simulink model "myTMSI"  (R2017b)
settings: Solver=FixedStepAuto  StartTime=0.0  StopTime=Inf  FixedStep=0.01  RelTol=1e-3
StopFcn:
  | [file,path] = uiputfile;
  | cd(path)
  | save(file, 'EMGdata', 'EMGcount', 'QuatAngle', 'Angles', 'Angles23', 'QuatAngle1')
  | cd ..
libraries: dspindex x16
settings Model: SimulationMode=external  ExtModeTrigDuration=50000  Creator=constantin  LastModifiedBy=root
settings DataIOCC: SaveFormat=Array
settings OptimizationCC: ExpressionDepthLimit=2147483647  LifeSpan=1
settings DebuggingCC: UnderspecifiedInitializationDetection=Classic  MergeDetectMultiDrivingBlocksExec=none  SolverPrmCheckMsg=warning  StateNameClashWarn=warning  SFUnexpectedBacktrackingDiag=warning  SFNoUnconditionalDefaultTransitionDiag=warning  SFExecutionAtInitializationDiag=none
settings HardwareCC: ProdBitPerPointer=32  ProdBitPerSizeT=32  ProdBitPerPtrDiffT=32  ProdLargestAtomicFloat=None  ProdIntDivRoundTo=Undefined  ProdEndianess=Unspecified  ProdWordSize=32  ProdHWDeviceType=32-bit Generic
settings ModelReferenceCC: PropagateSignalLabelsOutOfModel=off
settings SFSimCC: MATLABDynamicMemAlloc=off
settings RTWCC: SystemTargetFile=ert_linux.tlc  MakeCommand=make_rtw OPTS=-DWITH_HW OPTIMIZATION_FLAGS=-O3  TemplateMakefile=ert_linux.tmf  Description=Linux Embedded Coder  TargetLang=C++
settings CodeAppCC: IgnoreCustomStorageClasses=off  CustomSymbolStrType=$N$R$M  StateflowObjectComments=on  InternalIdentifier=Classic
settings STFCustomTargetCC: ModelReferenceCompliant=off  CombineOutputUpdateFcns=on  ERTCustomFileBanners=on  SupportComplex=off  RemoveResetFunc=on  SupportVariableSizeSignals=on  MATLABClassNameForMDSCustomization=Simulink.SoftwareTarget.ERTCustomization  GRTInterface=off  SystemTargetFile=ert_linux.tlc
settings ERTTargetCC: MultiwordLength=2048  ModelReferenceCompliant=off  ParMdlRefBuildCompliant=off  CompOptLevelCompliant=off  ConcurrentExecutionCompliant=off  SupportComplex=off  SupportContinuousTime=on  SupportNonInlinedSFcns=on  SupportVariableSizeSignals=on  ModelStepFunctionPrototypeControlCompliant=off  CPPClassGenCompliant=off  UseToolchainInfoCompliant=off  ExtMode=on  ExtModeMexArgs='127.0.0.1' 1 17725  MultiInstanceErrorCode=None  ERTCustomFileTemplate=ert_linux_file_process.tlc  ConvertIfToSwitch=off  SuppressUnreachableDefaultCases=off
settings ConfigComp: CovMetricSettings=dw  CovHtmlReporting=on  CovSaveCumulativeToWorkspaceVar=on  CovSaveSingleToWorkspaceVar=on  CovExternalEMLEnable=off  CovSFcnEnable=off
settings SimscapeCC: SimscapeNormalizeSystem=off
settings ConfigurationSet: Description=SimMechanics 2G

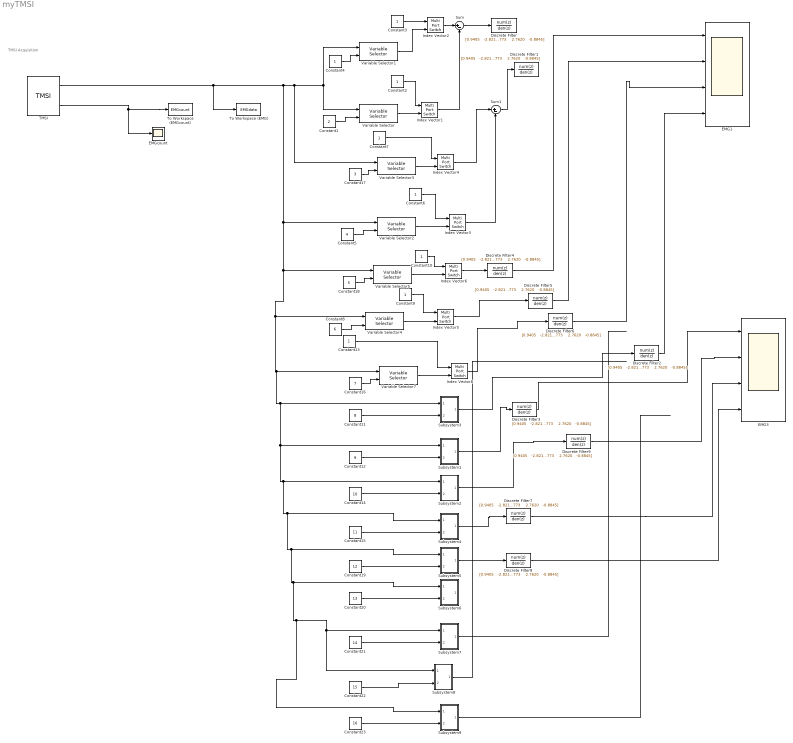
== system myTMSI ==
  note: TMSI Acquisition
  Constant1 : Constant  Value=2
  Constant{2..4,6..7,9..10,13} (8 alike) : Constant
  Constant11 : Constant  Value=8
  Constant12 : Constant  Value=9
  Constant14 : Constant  Value=10
  Constant15 : Constant  Value=11
  Constant16 : Constant  Value=7
  Constant17 : Constant  Value=3
  Constant18 : Constant  Value=5
  Constant19 : Constant  Value=12
  Constant20 : Constant  Value=13
  Constant21 : Constant  Value=14
  Constant22 : Constant  Value=15
  Constant23 : Constant  Value=16
  Constant5 : Constant  Value=4
  Constant8 : Constant  Value=6
  Discrete Filter : DiscreteFilter  Numerator=|  Denominator="[1.0000   -2.8773    2.7620   -0.8845]"
      | [0.9405   -2.8214    2.8214   -0.9405
      | ]
  Discrete Filter{1..9} (9 alike) : DiscreteFilter  Numerator="[0.9405   -2.8214    2.8214   -0.9405]"  Denominator="[1.0000   -2.8773    2.7620   -0.8845]"
  EMG1 : Scope  NumInputPorts=4
  EMG3 : Scope  NumInputPorts=4
  EMGcount : Scope
  Index Vector{1..6,8} (7 alike) : MultiPortSwitch  DataPortOrder=Zero-based contiguous  Inputs=1  zeroidx=on
  Subsystem1 : Subsystem
  Subsystem2 : Subsystem
  Subsystem3 : Subsystem
  Subsystem4 : Subsystem
  Subsystem5 : Subsystem
  Subsystem6 : Subsystem
  Subsystem7 : Subsystem
  Subsystem8 : Subsystem
  Subsystem9 : Subsystem
  Sum : Sum  Inputs=|+-
  Sum1 : Sum  Inputs=|+-
  TMSI : S-Function  FunctionName=TMSI  Parameters=uint16(frequency) int32(aux) int32(digital) int32(vectorsize) int32(ch)  SFunctionDeploymentMode=off  EnableBusSupport=off  mask{frequency=1, ch=[1 2 3 4 17 18 19 20 21 22 23 24 25 26 27 28], vectorsize=20, aux=29, digital=30}
      mask prompts: frequency "Please select a frequency"; ch "Please enter an array for channels e.g [17 29]"; vectorsize "Please enter the vector output size"; aux "Please enter the aux channel"; digital "Please enter digital channel"
      mask DialogControl DescTextVar Prompt: TMSI Block for EMG measurement
      mask Display:
      | disp('TMSI')
      | port_label('output', 1, 'data')
      | port_label('output', 2, 'status')
  To Workspace (EMG) : ToWorkspace  VariableName=EMGdata  SaveFormat=Structure With Time  SampleTime=-1
  To Workspace (EMGcount) : ToWorkspace  VariableName=EMGcount  SaveFormat=Structure With Time  SampleTime=-1
  Variable Selector{,1..5,7} (7 alike) : dspindex/Variable Selector  NumInputs=1  rowsOrCols=Rows  IdxMode=Variable  Elements=[1 3]  ZerOneIdxMode=One-based  errmode=Clip Index  FillMode=on  FillValues=0
  wires:
  TMSI/2 -> To Workspace (EMGcount)/1, EMGcount/1
  Constant1/1 -> Variable Selector/2
  Variable Selector/1 -> Index Vector1/2
  Constant2/1 -> Index Vector1/1
  Variable Selector1/1 -> Index Vector2/2
  Constant3/1 -> Index Vector2/1
  Constant4/1 -> Variable Selector1/2
  Variable Selector2/1 -> Index Vector3/2
  Constant6/1 -> Index Vector3/1
  Variable Selector3/1 -> Index Vector4/2
  Constant7/1 -> Index Vector4/1
  Constant5/1 -> Variable Selector2/2
  Constant17/1 -> Variable Selector3/2
  Index Vector6/1 -> Discrete Filter4/1
  Variable Selector4/1 -> Index Vector5/2
  Constant9/1 -> Index Vector5/1
  Variable Selector5/1 -> Index Vector6/2
  Constant10/1 -> Index Vector6/1
  Constant8/1 -> Variable Selector4/2
  Constant18/1 -> Variable Selector5/2
  Index Vector5/1 -> Discrete Filter5/1
  Index Vector8/1 -> Discrete Filter6/1
  Variable Selector7/1 -> Index Vector8/2
  Constant13/1 -> Index Vector8/1
  Constant16/1 -> Variable Selector7/2
  Index Vector4/1 -> Sum1/1
  Index Vector3/1 -> Sum1/2
  TMSI/1 -> To Workspace (EMG)/1, Subsystem3/1(In1), Subsystem9/1(In1), Subsystem7/1(In1), Subsystem8/1(In1), Subsystem6/1(In1), Subsystem5/1(In1), Subsystem4/1(In1), Subsystem2/1(In1), Subsystem1/1(In1), Variable Selector7/1, Variable Selector4/1, Variable Selector5/1, Variable Selector2/1, Variable Selector3/1, Variable Selector1/1, Variable Selector/1
  Index Vector2/1 -> Sum/1
  Index Vector1/1 -> Sum/2
  Sum/1 -> Discrete Filter/1
  Sum1/1 -> Discrete Filter1/1
  Discrete Filter4/1 -> EMG1/1
  Discrete Filter5/1 -> EMG1/2
  Discrete Filter6/1 -> EMG1/3
  Constant11/1 -> Subsystem3/2(In2)
  Subsystem3/1(Out1) -> Discrete Filter2/1
  Constant12/1 -> Subsystem1/2(In2)
  Constant14/1 -> Subsystem2/2(In2)
  Constant19/1 -> Subsystem5/2(In2)
  Constant15/1 -> Subsystem4/2(In2)
  Constant20/1 -> Subsystem6/2(In2)
  Constant21/1 -> Subsystem7/2(In2)
  Constant22/1 -> Subsystem8/2(In2)
  Constant23/1 -> Subsystem9/2(In2)
  Subsystem7/1(Out1) -> ?
  Subsystem8/1(Out1) -> ?
  Subsystem9/1(Out1) -> ?
  Discrete Filter2/1 -> EMG1/4
  Subsystem1/1(Out1) -> Discrete Filter3/1
  Discrete Filter3/1 -> EMG3/1
  Subsystem2/1(Out1) -> Discrete Filter9/1
  Subsystem4/1(Out1) -> Discrete Filter7/1
  Subsystem5/1(Out1) -> Discrete Filter8/1
  Discrete Filter9/1 -> EMG3/2
  Discrete Filter7/1 -> EMG3/3
  Discrete Filter8/1 -> EMG3/4

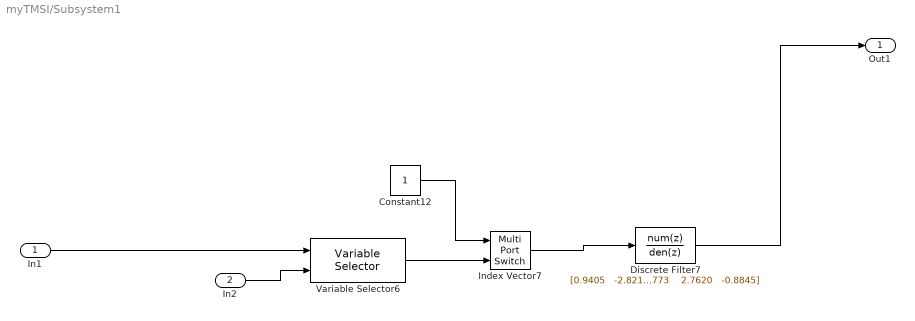
== system myTMSI/Subsystem1 ==
  In1 : Inport
  In2 : Inport  Port=2
  Constant12 : Constant
  Discrete Filter7 : DiscreteFilter  Numerator="[0.9405   -2.8214    2.8214   -0.9405]"  Denominator="[1.0000   -2.8773    2.7620   -0.8845]"
  Index Vector7 : MultiPortSwitch  DataPortOrder=Zero-based contiguous  Inputs=1  zeroidx=on
  Variable Selector6 : dspindex/Variable Selector  NumInputs=1  rowsOrCols=Rows  IdxMode=Variable  Elements=[1 3]  ZerOneIdxMode=One-based  errmode=Clip Index  FillMode=on  FillValues=0
  Out1 : Outport
  wires:
  In1/1 -> Variable Selector6/1
  Discrete Filter7/1 -> Out1/1
  Variable Selector6/1 -> Index Vector7/2
  Constant12/1 -> Index Vector7/1
  In2/1 -> Variable Selector6/2
  Index Vector7/1 -> Discrete Filter7/1

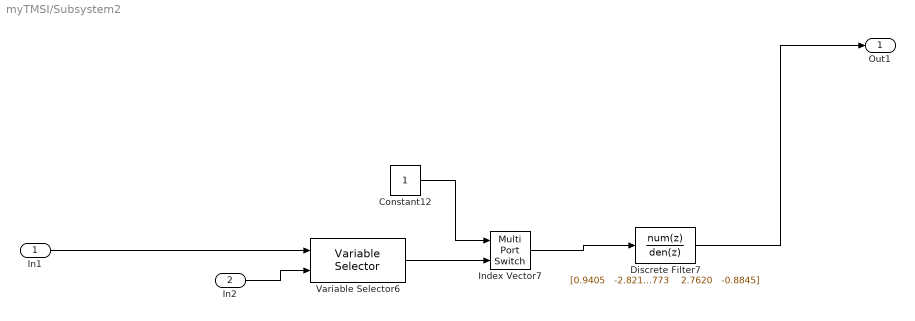
== system myTMSI/Subsystem2 ==
  In1 : Inport
  In2 : Inport  Port=2
  Constant12 : Constant
  Discrete Filter7 : DiscreteFilter  Numerator="[0.9405   -2.8214    2.8214   -0.9405]"  Denominator="[1.0000   -2.8773    2.7620   -0.8845]"
  Index Vector7 : MultiPortSwitch  DataPortOrder=Zero-based contiguous  Inputs=1  zeroidx=on
  Variable Selector6 : dspindex/Variable Selector  NumInputs=1  rowsOrCols=Rows  IdxMode=Variable  Elements=[1 3]  ZerOneIdxMode=One-based  errmode=Clip Index  FillMode=on  FillValues=0
  Out1 : Outport
  wires:
  In1/1 -> Variable Selector6/1
  Discrete Filter7/1 -> Out1/1
  Variable Selector6/1 -> Index Vector7/2
  Constant12/1 -> Index Vector7/1
  In2/1 -> Variable Selector6/2
  Index Vector7/1 -> Discrete Filter7/1

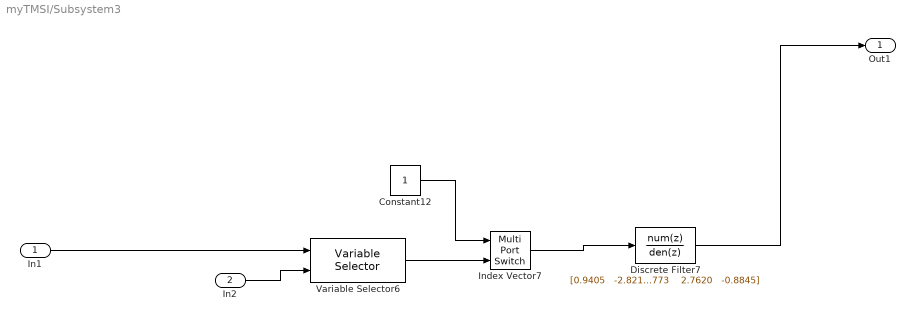
== system myTMSI/Subsystem3 ==
  In1 : Inport
  In2 : Inport  Port=2
  Constant12 : Constant
  Discrete Filter7 : DiscreteFilter  Numerator="[0.9405   -2.8214    2.8214   -0.9405]"  Denominator="[1.0000   -2.8773    2.7620   -0.8845]"
  Index Vector7 : MultiPortSwitch  DataPortOrder=Zero-based contiguous  Inputs=1  zeroidx=on
  Variable Selector6 : dspindex/Variable Selector  NumInputs=1  rowsOrCols=Rows  IdxMode=Variable  Elements=[1 3]  ZerOneIdxMode=One-based  errmode=Clip Index  FillMode=on  FillValues=0
  Out1 : Outport
  wires:
  In1/1 -> Variable Selector6/1
  Discrete Filter7/1 -> Out1/1
  Variable Selector6/1 -> Index Vector7/2
  Constant12/1 -> Index Vector7/1
  In2/1 -> Variable Selector6/2
  Index Vector7/1 -> Discrete Filter7/1

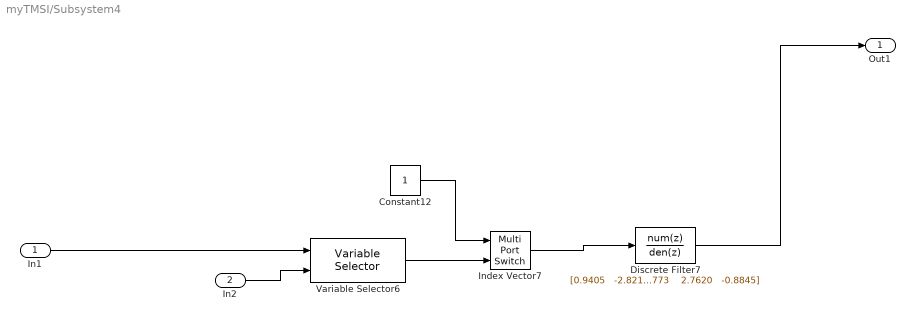
== system myTMSI/Subsystem4 ==
  In1 : Inport
  In2 : Inport  Port=2
  Constant12 : Constant
  Discrete Filter7 : DiscreteFilter  Numerator="[0.9405   -2.8214    2.8214   -0.9405]"  Denominator="[1.0000   -2.8773    2.7620   -0.8845]"
  Index Vector7 : MultiPortSwitch  DataPortOrder=Zero-based contiguous  Inputs=1  zeroidx=on
  Variable Selector6 : dspindex/Variable Selector  NumInputs=1  rowsOrCols=Rows  IdxMode=Variable  Elements=[1 3]  ZerOneIdxMode=One-based  errmode=Clip Index  FillMode=on  FillValues=0
  Out1 : Outport
  wires:
  In1/1 -> Variable Selector6/1
  Discrete Filter7/1 -> Out1/1
  Variable Selector6/1 -> Index Vector7/2
  Constant12/1 -> Index Vector7/1
  In2/1 -> Variable Selector6/2
  Index Vector7/1 -> Discrete Filter7/1

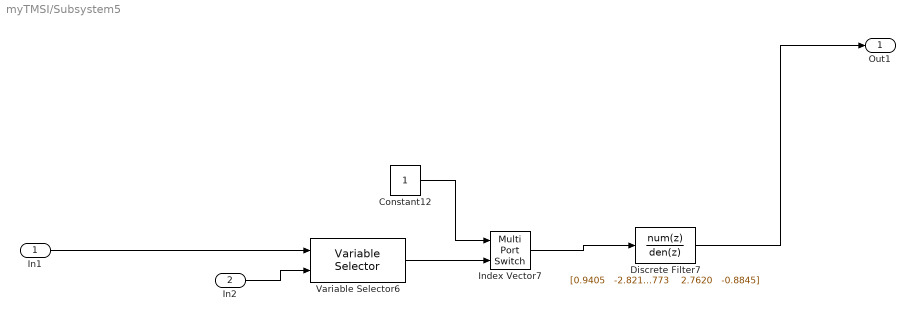
== system myTMSI/Subsystem5 ==
  In1 : Inport
  In2 : Inport  Port=2
  Constant12 : Constant
  Discrete Filter7 : DiscreteFilter  Numerator="[0.9405   -2.8214    2.8214   -0.9405]"  Denominator="[1.0000   -2.8773    2.7620   -0.8845]"
  Index Vector7 : MultiPortSwitch  DataPortOrder=Zero-based contiguous  Inputs=1  zeroidx=on
  Variable Selector6 : dspindex/Variable Selector  NumInputs=1  rowsOrCols=Rows  IdxMode=Variable  Elements=[1 3]  ZerOneIdxMode=One-based  errmode=Clip Index  FillMode=on  FillValues=0
  Out1 : Outport
  wires:
  In1/1 -> Variable Selector6/1
  Discrete Filter7/1 -> Out1/1
  Variable Selector6/1 -> Index Vector7/2
  Constant12/1 -> Index Vector7/1
  In2/1 -> Variable Selector6/2
  Index Vector7/1 -> Discrete Filter7/1

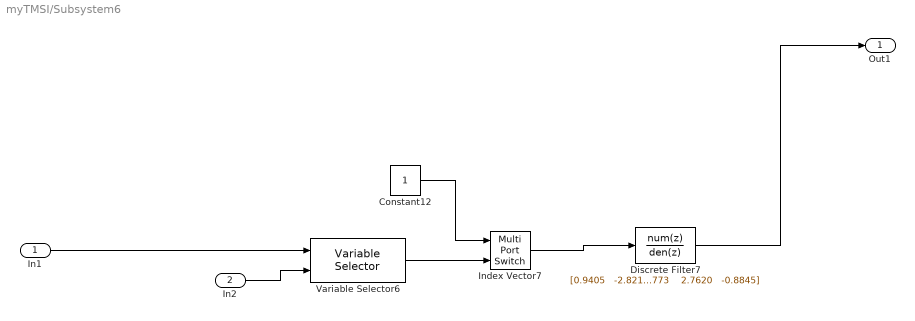
== system myTMSI/Subsystem6 ==
  In1 : Inport
  In2 : Inport  Port=2
  Constant12 : Constant
  Discrete Filter7 : DiscreteFilter  Numerator="[0.9405   -2.8214    2.8214   -0.9405]"  Denominator="[1.0000   -2.8773    2.7620   -0.8845]"
  Index Vector7 : MultiPortSwitch  DataPortOrder=Zero-based contiguous  Inputs=1  zeroidx=on
  Variable Selector6 : dspindex/Variable Selector  NumInputs=1  rowsOrCols=Rows  IdxMode=Variable  Elements=[1 3]  ZerOneIdxMode=One-based  errmode=Clip Index  FillMode=on  FillValues=0
  Out1 : Outport
  wires:
  In1/1 -> Variable Selector6/1
  Discrete Filter7/1 -> Out1/1
  Variable Selector6/1 -> Index Vector7/2
  Constant12/1 -> Index Vector7/1
  In2/1 -> Variable Selector6/2
  Index Vector7/1 -> Discrete Filter7/1

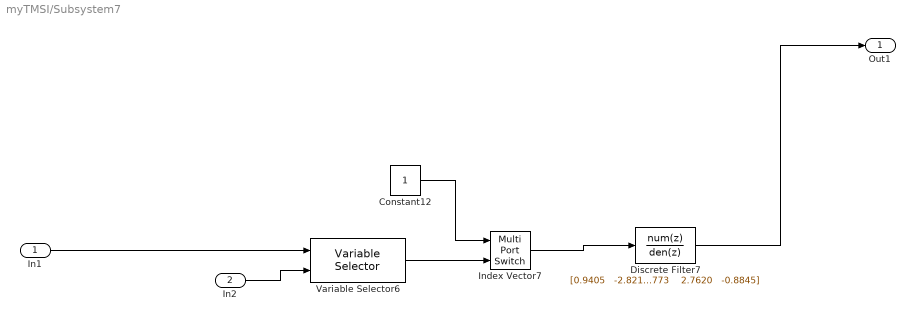
== system myTMSI/Subsystem7 ==
  In1 : Inport
  In2 : Inport  Port=2
  Constant12 : Constant
  Discrete Filter7 : DiscreteFilter  Numerator="[0.9405   -2.8214    2.8214   -0.9405]"  Denominator="[1.0000   -2.8773    2.7620   -0.8845]"
  Index Vector7 : MultiPortSwitch  DataPortOrder=Zero-based contiguous  Inputs=1  zeroidx=on
  Variable Selector6 : dspindex/Variable Selector  NumInputs=1  rowsOrCols=Rows  IdxMode=Variable  Elements=[1 3]  ZerOneIdxMode=One-based  errmode=Clip Index  FillMode=on  FillValues=0
  Out1 : Outport
  wires:
  In1/1 -> Variable Selector6/1
  Discrete Filter7/1 -> Out1/1
  Variable Selector6/1 -> Index Vector7/2
  Constant12/1 -> Index Vector7/1
  In2/1 -> Variable Selector6/2
  Index Vector7/1 -> Discrete Filter7/1

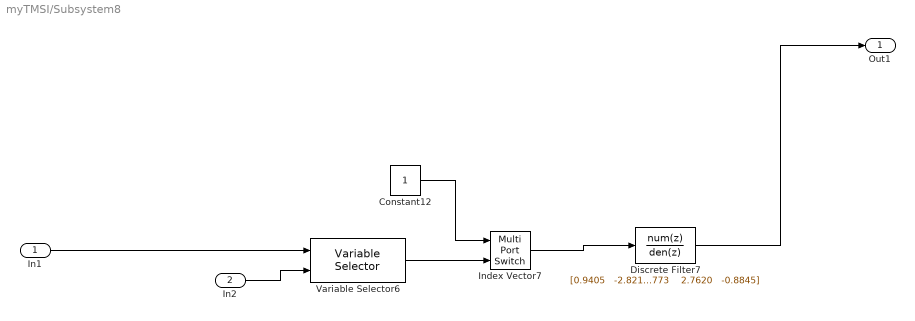
== system myTMSI/Subsystem8 ==
  In1 : Inport
  In2 : Inport  Port=2
  Constant12 : Constant
  Discrete Filter7 : DiscreteFilter  Numerator="[0.9405   -2.8214    2.8214   -0.9405]"  Denominator="[1.0000   -2.8773    2.7620   -0.8845]"
  Index Vector7 : MultiPortSwitch  DataPortOrder=Zero-based contiguous  Inputs=1  zeroidx=on
  Variable Selector6 : dspindex/Variable Selector  NumInputs=1  rowsOrCols=Rows  IdxMode=Variable  Elements=[1 3]  ZerOneIdxMode=One-based  errmode=Clip Index  FillMode=on  FillValues=0
  Out1 : Outport
  wires:
  In1/1 -> Variable Selector6/1
  Discrete Filter7/1 -> Out1/1
  Variable Selector6/1 -> Index Vector7/2
  Constant12/1 -> Index Vector7/1
  In2/1 -> Variable Selector6/2
  Index Vector7/1 -> Discrete Filter7/1

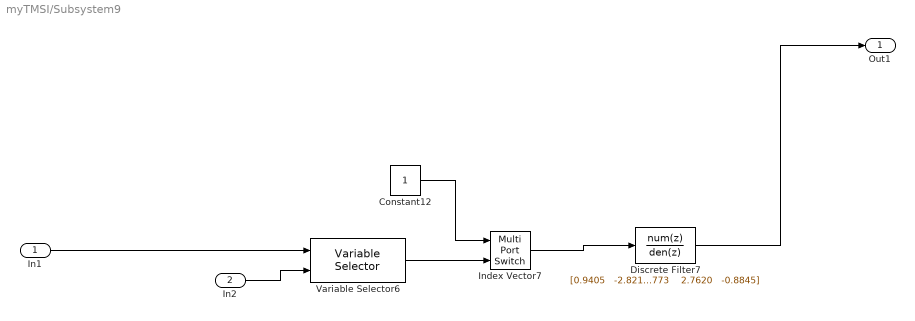
== system myTMSI/Subsystem9 ==
  In1 : Inport
  In2 : Inport  Port=2
  Constant12 : Constant
  Discrete Filter7 : DiscreteFilter  Numerator="[0.9405   -2.8214    2.8214   -0.9405]"  Denominator="[1.0000   -2.8773    2.7620   -0.8845]"
  Index Vector7 : MultiPortSwitch  DataPortOrder=Zero-based contiguous  Inputs=1  zeroidx=on
  Variable Selector6 : dspindex/Variable Selector  NumInputs=1  rowsOrCols=Rows  IdxMode=Variable  Elements=[1 3]  ZerOneIdxMode=One-based  errmode=Clip Index  FillMode=on  FillValues=0
  Out1 : Outport
  wires:
  In1/1 -> Variable Selector6/1
  Discrete Filter7/1 -> Out1/1
  Variable Selector6/1 -> Index Vector7/2
  Constant12/1 -> Index Vector7/1
  In2/1 -> Variable Selector6/2
  Index Vector7/1 -> Discrete Filter7/1
